simulink model "V2x_TC_CarBreakdownWarning_cs"  (Simulink 7.6)
settings: Solver=ode5  SolverMode=SingleTasking  StartTime=0.0  StopTime=18  FixedStep=1/100  RelTol=1e-3
PreLoadFcn:
  | check_NUTS_defined;
  | 
  | assignin('base',['model_closed_' bdroot],false);addpath('../includes_V2x');
InitFcn:
  | PreScanExperimentInitFcn(bdroot)
StopFcn:
  | PreScanExperimentStopFcn(bdroot)
undefined symbols (not defined in the file or in its folder): acceleration, actorID, actorType, DiscIntNeverNeededParam, GPS_alt, GPS_lat, GPS_long, intmax, lightBarInUse, messageID, Newton, publicActorType, Raphson, rotZ, sigbuilder_block, sireneInUse, trafficLightPriority, turnAdvice, velocity, x_ini_VRML, y_ini_VRML, yawRate, z_ini_VRML
libraries: simulink x61, PreScanSimulinkLibrary x19, PreScanUsefulBlocks x7, simulink_extras x1
(part 10 of 10)

== system V2x_TC_CarBreakdownWarning_cs/Audi_A8_1/vehicle CAM generator/CAM generation/maybe/If Action Subsystem ==
  x [m] : Inport
  y [m] : Inport  Port=2
  z [m] : Inport  Port=3
  rotZ [deg] : Inport  Port=4
  velocity [m/s] : Inport  Port=5
  Action Port : ActionPort  PropagateVarSize=During execution  ActionType=then
  Constant : Constant
  Data Store Write : DataStoreWrite  DataStoreName=CAM_velocity
  Data Store Write1 : DataStoreWrite  DataStoreName=CAM_heading
  Data Store Write2 : DataStoreWrite  DataStoreName=CAM_x
  Data Store Write3 : DataStoreWrite  DataStoreName=CAM_y
  Data Store Write4 : DataStoreWrite  DataStoreName=CAM_z
  Data Store Write5 : DataStoreWrite  DataStoreName=CAM_time
  Digital Clock1 : DigitalClock  SampleTime=0.01
  Out1 : Outport  InitialOutput=0
  wires:
  Constant/1 -> Out1/1
  velocity [m/s]/1 -> Data Store Write/1
  rotZ [deg]/1 -> Data Store Write1/1
  x [m]/1 -> Data Store Write2/1
  y [m]/1 -> Data Store Write3/1
  z [m]/1 -> Data Store Write4/1
  Digital Clock1/1 -> Data Store Write5/1

== system V2x_TC_CarBreakdownWarning_cs/Audi_A8_1/vehicle CAM generator/CAM generation/maybe/If Action Subsystem1 ==
  Action Port : ActionPort  PropagateVarSize=During execution  ActionType=else
  Constant : Constant  Value=0
  Out1 : Outport  InitialOutput=0
  wires:
  Constant/1 -> Out1/1

== system V2x_TC_CarBreakdownWarning_cs/BMW_X5_1/Trajectories/Traj2State1/Traj2State2/MuxState ==
  x [m] : Inport
  y [m] : Inport  Port=2
  z [m] : Inport  Port=3
  dx [m/s] : Inport  Port=4
  dy [m/s] : Inport  Port=5
  dz [m/s] : Inport  Port=6
  R [rad] : Inport  Port=7
  P [rad] : Inport  Port=8
  Y [rad] : Inport  Port=9
  Mux : Mux  Inputs=9
  state : Outport
  wires:
  z [m]/1 -> Mux/3
  y [m]/1 -> Mux/2
  x [m]/1 -> Mux/1
  Y [rad]/1 -> Mux/9
  P [rad]/1 -> Mux/8
  R [rad]/1 -> Mux/7
  dz [m/s]/1 -> Mux/6
  dy [m/s]/1 -> Mux/5
  dx [m/s]/1 -> Mux/4
  Mux/1 -> state/1

== system V2x_TC_CarBreakdownWarning_cs/BMW_X5_1/Trajectories/Traj2State1/Traj2State2/Traj2MuxState_Ext ==
  Traj : Inport
  Terminator{1..9} (9 alike) : Terminator
  demux : Subsystem
  x [m] : Outport
  y [m] : Outport  Port=2
  z [m] : Outport  Port=3
  dx [m/s] : Outport  Port=4
  dy [m/s] : Outport  Port=5
  dz [m/s] : Outport  Port=6
  R [rad] : Outport  Port=7
  P [rad] : Outport  Port=8
  Y [rad] : Outport  Port=9
  wires:
  demux/9(Y) -> Y [rad]/1
  demux/7(R) -> R [rad]/1
  demux/5(vely) -> dy [m/s]/1
  demux/4(velx) -> dx [m/s]/1
  demux/10(velR) -> Terminator4/1
  demux/11(velP) -> Terminator5/1
  demux/12(velY) -> Terminator1/1
  demux/13(accx) -> Terminator8/1
  demux/14(accy) -> Terminator9/1
  demux/15(accz) -> Terminator7/1
  demux/18(accY) -> Terminator2/1
  demux/16(accR) -> Terminator3/1
  demux/17(accP) -> Terminator6/1
  demux/3(z) -> z [m]/1
  Traj/1 -> demux/1(traj)
  demux/6(velz) -> dz [m/s]/1
  demux/1(x) -> x [m]/1
  demux/2(y) -> y [m]/1
  demux/8(P) -> P [rad]/1

== system V2x_TC_CarBreakdownWarning_cs/BMW_X5_1/vehicle CAM generator/CAM generation/maybe/If Action Subsystem ==
  x [m] : Inport
  y [m] : Inport  Port=2
  z [m] : Inport  Port=3
  rotZ [deg] : Inport  Port=4
  velocity [m/s] : Inport  Port=5
  Action Port : ActionPort  PropagateVarSize=During execution  ActionType=then
  Constant : Constant
  Data Store Write : DataStoreWrite  DataStoreName=CAM_velocity
  Data Store Write1 : DataStoreWrite  DataStoreName=CAM_heading
  Data Store Write2 : DataStoreWrite  DataStoreName=CAM_x
  Data Store Write3 : DataStoreWrite  DataStoreName=CAM_y
  Data Store Write4 : DataStoreWrite  DataStoreName=CAM_z
  Data Store Write5 : DataStoreWrite  DataStoreName=CAM_time
  Digital Clock1 : DigitalClock  SampleTime=0.01
  Out1 : Outport  InitialOutput=0
  wires:
  Constant/1 -> Out1/1
  velocity [m/s]/1 -> Data Store Write/1
  rotZ [deg]/1 -> Data Store Write1/1
  x [m]/1 -> Data Store Write2/1
  y [m]/1 -> Data Store Write3/1
  z [m]/1 -> Data Store Write4/1
  Digital Clock1/1 -> Data Store Write5/1

== system V2x_TC_CarBreakdownWarning_cs/BMW_X5_1/vehicle CAM generator/CAM generation/maybe/If Action Subsystem1 ==
  Action Port : ActionPort  PropagateVarSize=During execution  ActionType=else
  Constant : Constant  Value=0
  Out1 : Outport  InitialOutput=0
  wires:
  Constant/1 -> Out1/1

== system V2x_TC_CarBreakdownWarning_cs/Fiat_Bravo_1/Trajectories/Traj2State1/Traj2State2/MuxState ==
  x [m] : Inport
  y [m] : Inport  Port=2
  z [m] : Inport  Port=3
  dx [m/s] : Inport  Port=4
  dy [m/s] : Inport  Port=5
  dz [m/s] : Inport  Port=6
  R [rad] : Inport  Port=7
  P [rad] : Inport  Port=8
  Y [rad] : Inport  Port=9
  Mux : Mux  Inputs=9
  state : Outport
  wires:
  z [m]/1 -> Mux/3
  y [m]/1 -> Mux/2
  x [m]/1 -> Mux/1
  Y [rad]/1 -> Mux/9
  P [rad]/1 -> Mux/8
  R [rad]/1 -> Mux/7
  dz [m/s]/1 -> Mux/6
  dy [m/s]/1 -> Mux/5
  dx [m/s]/1 -> Mux/4
  Mux/1 -> state/1

== system V2x_TC_CarBreakdownWarning_cs/Fiat_Bravo_1/Trajectories/Traj2State1/Traj2State2/Traj2MuxState_Ext ==
  Traj : Inport
  Terminator{1..9} (9 alike) : Terminator
  demux : Subsystem
  x [m] : Outport
  y [m] : Outport  Port=2
  z [m] : Outport  Port=3
  dx [m/s] : Outport  Port=4
  dy [m/s] : Outport  Port=5
  dz [m/s] : Outport  Port=6
  R [rad] : Outport  Port=7
  P [rad] : Outport  Port=8
  Y [rad] : Outport  Port=9
  wires:
  demux/9(Y) -> Y [rad]/1
  demux/7(R) -> R [rad]/1
  demux/5(vely) -> dy [m/s]/1
  demux/4(velx) -> dx [m/s]/1
  demux/10(velR) -> Terminator4/1
  demux/11(velP) -> Terminator5/1
  demux/12(velY) -> Terminator1/1
  demux/13(accx) -> Terminator8/1
  demux/14(accy) -> Terminator9/1
  demux/15(accz) -> Terminator7/1
  demux/18(accY) -> Terminator2/1
  demux/16(accR) -> Terminator3/1
  demux/17(accP) -> Terminator6/1
  demux/3(z) -> z [m]/1
  Traj/1 -> demux/1(traj)
  demux/6(velz) -> dz [m/s]/1
  demux/1(x) -> x [m]/1
  demux/2(y) -> y [m]/1
  demux/8(P) -> P [rad]/1

== system V2x_TC_CarBreakdownWarning_cs/Fiat_Bravo_1/vehicle CAM generator/CAM generation/maybe/If Action Subsystem ==
  x [m] : Inport
  y [m] : Inport  Port=2
  z [m] : Inport  Port=3
  rotZ [deg] : Inport  Port=4
  velocity [m/s] : Inport  Port=5
  Action Port : ActionPort  PropagateVarSize=During execution  ActionType=then
  Constant : Constant
  Data Store Write : DataStoreWrite  DataStoreName=CAM_velocity
  Data Store Write1 : DataStoreWrite  DataStoreName=CAM_heading
  Data Store Write2 : DataStoreWrite  DataStoreName=CAM_x
  Data Store Write3 : DataStoreWrite  DataStoreName=CAM_y
  Data Store Write4 : DataStoreWrite  DataStoreName=CAM_z
  Data Store Write5 : DataStoreWrite  DataStoreName=CAM_time
  Digital Clock1 : DigitalClock  SampleTime=0.01
  Out1 : Outport  InitialOutput=0
  wires:
  Constant/1 -> Out1/1
  velocity [m/s]/1 -> Data Store Write/1
  rotZ [deg]/1 -> Data Store Write1/1
  x [m]/1 -> Data Store Write2/1
  y [m]/1 -> Data Store Write3/1
  z [m]/1 -> Data Store Write4/1
  Digital Clock1/1 -> Data Store Write5/1

== system V2x_TC_CarBreakdownWarning_cs/Fiat_Bravo_1/vehicle CAM generator/CAM generation/maybe/If Action Subsystem1 ==
  Action Port : ActionPort  PropagateVarSize=During execution  ActionType=else
  Constant : Constant  Value=0
  Out1 : Outport  InitialOutput=0
  wires:
  Constant/1 -> Out1/1

== system V2x_TC_CarBreakdownWarning_cs/Toyota_Previa_1/vehicle CAM generator/CAM generation/maybe/If Action Subsystem ==
  x [m] : Inport
  y [m] : Inport  Port=2
  z [m] : Inport  Port=3
  rotZ [deg] : Inport  Port=4
  velocity [m/s] : Inport  Port=5
  Action Port : ActionPort  PropagateVarSize=During execution  ActionType=then
  Constant : Constant
  Data Store Write : DataStoreWrite  DataStoreName=CAM_velocity
  Data Store Write1 : DataStoreWrite  DataStoreName=CAM_heading
  Data Store Write2 : DataStoreWrite  DataStoreName=CAM_x
  Data Store Write3 : DataStoreWrite  DataStoreName=CAM_y
  Data Store Write4 : DataStoreWrite  DataStoreName=CAM_z
  Data Store Write5 : DataStoreWrite  DataStoreName=CAM_time
  Digital Clock1 : DigitalClock  SampleTime=0.01
  Out1 : Outport  InitialOutput=0
  wires:
  Constant/1 -> Out1/1
  velocity [m/s]/1 -> Data Store Write/1
  rotZ [deg]/1 -> Data Store Write1/1
  x [m]/1 -> Data Store Write2/1
  y [m]/1 -> Data Store Write3/1
  z [m]/1 -> Data Store Write4/1
  Digital Clock1/1 -> Data Store Write5/1

== system V2x_TC_CarBreakdownWarning_cs/Toyota_Previa_1/vehicle CAM generator/CAM generation/maybe/If Action Subsystem1 ==
  Action Port : ActionPort  PropagateVarSize=During execution  ActionType=else
  Constant : Constant  Value=0
  Out1 : Outport  InitialOutput=0
  wires:
  Constant/1 -> Out1/1

== system V2x_TC_CarBreakdownWarning_cs/Audi_A8_1/Traffic Controller/Intersection warning controller/Enabled Subsystem/Intersection/Closest crossing selection ==
  crossingType : Inport
  host GPS lat : Inport  Port=2
  host GPS long : Inport  Port=3
  host GPS alt : Inport  Port=4
  GPS lat : Inport  Port=5
  GPS long : Inport  Port=6
  GPS alt : Inport  Port=7
  crossing detection range : Inport  Port=8
  GPS alt1 : InportShadow  Port=7
  GPS lat1 : InportShadow  Port=5
  GPS long1 : InportShadow  Port=6
  GPS to XYZ difference (vectorized) : Subsystem
  If : If  NumInputs=2  IfExpression=u1 ~= u2
  If Action Subsystem : Subsystem  TreatAsAtomicUnit=on
  If Action Subsystem1 : Subsystem  TreatAsAtomicUnit=on
  Logical Operator : Logic  AllPortsSameDT=off  OutDataTypeStr=boolean
  Merge : Merge
  Merge1 : Merge
  Merge2 : Merge
  MinMax : MinMax
  Product : Product  RndMeth=Zero
  Relational Operator : RelationalOperator  Operator=<  OutDataTypeStr=boolean
  Switch : Switch  Criteria=u2 > Threshold
  crossing GPS lat : Outport
  crossing GPS long : Outport  Port=2
  crossing GPS alt : Outport  Port=3
  wires:
  GPS to XYZ difference (vectorized)/1(dist_sq) -> Relational Operator/1, Switch/1, If Action Subsystem/2(dist_sq)
  crossing detection range/1 -> Product/2, Product/1
  Product/1 -> Relational Operator/2, Switch/3, If/2
  Relational Operator/1 -> Logical Operator/1
  crossingType/1 -> Logical Operator/2
  Logical Operator/1 -> Switch/2
  Switch/1 -> MinMax/1
  MinMax/1 -> If Action Subsystem/1(min), If/1
  host GPS lat/1 -> GPS to XYZ difference (vectorized)/1(hostLat)
  host GPS long/1 -> GPS to XYZ difference (vectorized)/2(hostLong)
  host GPS alt/1 -> GPS to XYZ difference (vectorized)/3(hostAlt)
  GPS lat/1 -> GPS to XYZ difference (vectorized)/4(lat)
  GPS long/1 -> GPS to XYZ difference (vectorized)/5(long)
  GPS alt/1 -> GPS to XYZ difference (vectorized)/6(alt)
  If/1 -> If Action Subsystem/Action
  If/2 -> If Action Subsystem1/Action
  GPS lat1/1 -> If Action Subsystem/3(GPS lat1)
  GPS long1/1 -> If Action Subsystem/4(GPS long1)
  GPS alt1/1 -> If Action Subsystem/5(GPS alt1)
  If Action Subsystem/1(GPS lat) -> Merge/1
  If Action Subsystem/2(GPS long) -> Merge2/1
  If Action Subsystem/3(GPS alt) -> Merge1/1
  If Action Subsystem1/1(GPS lat) -> Merge/2
  If Action Subsystem1/2(GPS long) -> Merge2/2
  If Action Subsystem1/3(GPS alt) -> Merge1/2
  Merge2/1 -> crossing GPS long/1
  Merge/1 -> crossing GPS lat/1
  Merge1/1 -> crossing GPS alt/1

== system V2x_TC_CarBreakdownWarning_cs/Audi_A8_1/Traffic Controller/Intersection warning controller/Enabled Subsystem/Intersection/GPS to XYZ difference (vectorized) ==
  hostLat : Inport
  hostLong : Inport  Port=2
  hostAlt : Inport  Port=3
  lat : Inport  Port=4
  long : Inport  Port=5
  alt : Inport  Port=6
  Add : Sum  Inputs=+-
  Add1 : Sum  Inputs=+-
  Add2 : Sum  Inputs=+-
  Product1 : Product  RndMeth=Zero
  Product2 : Product  RndMeth=Zero
  d2r : Gain  Gain=pi/180
  d2r1 : Gain  Gain=pi/180
  mean Earth radius (latitudal) : Constant  Value=6335439.8775
  mean Earth radius (longitudal) : Constant  Value=6378137.55
  dX : Outport
  dY : Outport  Port=2
  dZ : Outport  Port=3
  wires:
  lat/1 -> Add/1
  hostLat/1 -> Add/2
  long/1 -> Add1/1
  hostLong/1 -> Add1/2
  alt/1 -> Add2/1
  hostAlt/1 -> Add2/2
  Add/1 -> d2r/1
  Add1/1 -> d2r1/1
  d2r/1 -> Product2/1
  d2r1/1 -> Product1/1
  mean Earth radius (longitudal)/1 -> Product1/2
  mean Earth radius (latitudal)/1 -> Product2/2
  Product2/1 -> dY/1
  Product1/1 -> dX/1
  Add2/1 -> dZ/1

== system V2x_TC_CarBreakdownWarning_cs/Audi_A8_1/Traffic Controller/Intersection warning controller/Enabled Subsystem/Intersection/Intersection collision warning controller ==
  actorType : Inport
  hostTurnAdvice : Inport  Port=2
  crossing detection range : Inport  Port=3
  target intention : Inport  Port=4
  target velocity : Inport  Port=5
  target range : Inport  Port=6
  target angle : Inport  Port=7
  target heading : Inport  Port=8
  For Each Subsystem : Subsystem  TreatAsAtomicUnit=on
  Logical Operator : Logic  Operator=OR  Inputs=1  AllPortsSameDT=off  OutDataTypeStr=boolean
  Logical Operator1 : Logic  Operator=OR  Inputs=1  AllPortsSameDT=off  OutDataTypeStr=boolean
  Logical Operator2 : Logic  Operator=OR  Inputs=1  AllPortsSameDT=off  OutDataTypeStr=boolean
  host intention translation : Subsystem
  warning left lane : Outport
  warning straight lane : Outport  Port=2
  warning right lane : Outport  Port=3
  wires:
  hostTurnAdvice/1 -> host intention translation/1(host intention)
  For Each Subsystem/1(warning left lane) -> Logical Operator/1
  For Each Subsystem/2(warning straight lane) -> Logical Operator1/1
  For Each Subsystem/3(warning right lane) -> Logical Operator2/1
  actorType/1 -> For Each Subsystem/1(actorType)
  host intention translation/1(WM) -> For Each Subsystem/2(WM)
  crossing detection range/1 -> For Each Subsystem/3(Rcross)
  target range/1 -> For Each Subsystem/4(target range)
  target angle/1 -> For Each Subsystem/5(target angle)
  target intention/1 -> For Each Subsystem/6(target intention)
  target heading/1 -> For Each Subsystem/7(target heading)
  Logical Operator/1 -> warning left lane/1
  Logical Operator1/1 -> warning straight lane/1
  Logical Operator2/1 -> warning right lane/1
  target velocity/1 -> For Each Subsystem/8(targetVelocity)

== system V2x_TC_CarBreakdownWarning_cs/Audi_A8_1/Traffic Controller/Intersection warning controller/Enabled Subsystem/Intersection/cartesian 2 cylindrical ==
  dX : Inport
  dY : Inport  Port=2
  hostRotZ : Inport  Port=3
  Add : Sum  Inputs=+-
  Complex to Magnitude-Angle1 : ComplexToMagnitudeAngle
  Real-Imag to Complex1 : RealImagToComplex
  r2d : Gain  Gain=180/pi
  range : Outport
  angle : Outport  Port=2
  wires:
  Real-Imag to Complex1/1 -> Complex to Magnitude-Angle1/1
  dX/1 -> Real-Imag to Complex1/1
  Complex to Magnitude-Angle1/1 -> range/1  "range"
  dY/1 -> Real-Imag to Complex1/2
  Complex to Magnitude-Angle1/2 -> r2d/1  "angle"
  r2d/1 -> Add/1
  hostRotZ/1 -> Add/2
  Add/1 -> angle/1

== system V2x_TC_CarBreakdownWarning_cs/Audi_A8_1/Traffic Controller/Intersection warning controller/Enabled Subsystem/Intersection/relative heading ==
  rotZ : Inport
  hostRotZ : Inport  Port=2
  Add : Sum  Inputs=+-
  Constant : Constant  Value=360
  Math Function : Math  Operator=mod  SaturateOnIntegerOverflow=on
  dRotZ : Outport
  wires:
  Constant/1 -> Math Function/2
  rotZ/1 -> Add/1
  hostRotZ/1 -> Add/2
  Add/1 -> Math Function/1
  Math Function/1 -> dRotZ/1

== system V2x_TC_CarBreakdownWarning_cs/Audi_A8_1/Traffic Controller/Road accident detection controller/Compute distance to road accident/If Action Subsystem/GPS to distance ==
  hostLat : Inport
  hostLong : Inport  Port=2
  hostAlt : Inport  Port=3
  lat : Inport  Port=4
  long : Inport  Port=5
  alt : Inport  Port=6
  Add : Sum  Inputs=+-
  Add1 : Sum  Inputs=+-
  Add2 : Sum  Inputs=+-
  Add3 : Sum  Inputs=+++
  Product{,1..4} (5 alike) : Product  RndMeth=Zero
  Sqrt : Sqrt  AlgorithmType=Newton-Raphson  SaturateOnIntegerOverflow=on
  d2r : Gain  Gain=pi/180
  d2r1 : Gain  Gain=pi/180
  mean Earth radius (latitudal) : Constant  Value=6335439.8775
  mean Earth radius (longitudal) : Constant  Value=6378137.55
  dist : Outport
  wires:
  lat/1 -> Add/1
  hostLat/1 -> Add/2
  long/1 -> Add1/1
  hostLong/1 -> Add1/2
  alt/1 -> Add2/1
  hostAlt/1 -> Add2/2
  Add/1 -> d2r/1
  Add1/1 -> d2r1/1
  d2r/1 -> Product2/1
  d2r1/1 -> Product1/1
  mean Earth radius (longitudal)/1 -> Product1/2
  mean Earth radius (latitudal)/1 -> Product2/2
  Product2/1 -> Product/1, Product/2
  Product1/1 -> Product3/1, Product3/2
  Add2/1 -> Product4/2, Product4/1
  Product/1 -> Add3/1
  Product3/1 -> Add3/2
  Product4/1 -> Add3/3
  Add3/1 -> Sqrt/1
  Sqrt/1 -> dist/1

== system V2x_TC_CarBreakdownWarning_cs/Audi_A8_1/Traffic Controller/Traffic signs and  traffic lights controller/Enabled Subsystem/distance condition/If Action Subsystem ==
  d2 : Inport
  v2 : Inport  Port=2
  Action Port : ActionPort  PropagateVarSize=During execution  ActionType=then
  Divide : Product  Inputs=*/
  t2 : Outport
  wires:
  Divide/1 -> t2/1
  v2/1 -> Divide/2
  d2/1 -> Divide/1

== system V2x_TC_CarBreakdownWarning_cs/Audi_A8_1/Traffic Controller/Traffic signs and  traffic lights controller/Enabled Subsystem/distance condition/If Action Subsystem1 ==
  headway time : Inport
  d2 : Inport  Port=2
  Action Port : ActionPort  PropagateVarSize=During execution  ActionType=else
  Add : Sum
  Gain : Gain  Gain=0
  t2 : Outport
  wires:
  Add/1 -> t2/1
  headway time/1 -> Add/2
  Gain/1 -> Add/1
  d2/1 -> Gain/1

== system V2x_TC_CarBreakdownWarning_cs/Audi_A8_1/Traffic Controller/Traffic signs and  traffic lights controller/Enabled Subsystem/major object selection lights/If Action Subsystem ==
  cond : Inport
  messagesID : Inport  Port=2
  traffic lights priorities : Inport  Port=3
  Action Port : ActionPort  PropagateVarSize=During execution  ActionType=then
  Reshape1 : Reshape  OutputDimensionality=Column vector (2-D)
  Reshape2 : Reshape  OutputDimensionality=Column vector (2-D)
  Reshape3 : Reshape  OutputDimensionality=Column vector (2-D)
  Selector : Selector  NumberOfDimensions=2  InputPortWidth=3  IndexOptions=Index vector (port),Index vector (dialog)  Indices=[1 3],1  OutputSizes=1,1
  Selector1 : Selector  NumberOfDimensions=2  InputPortWidth=3  IndexOptions=Index vector (port),Index vector (dialog)  Indices=[1 3],1  OutputSizes=1,1
  While Iterator Subsystem : Subsystem  TreatAsAtomicUnit=on
  Message : Outport  InitialOutput=0
  Priority : Outport  Port=2  InitialOutput=0
  wires:
  Selector1/1 -> Priority/1
  Reshape3/1 -> Selector1/1
  traffic lights priorities/1 -> Reshape3/1
  messagesID/1 -> Reshape2/1
  While Iterator Subsystem/1(idx) -> Selector1/2, Selector/2
  Reshape2/1 -> Selector/1
  Reshape1/1 -> While Iterator Subsystem/1(cond)
  Selector/1 -> Message/1
  cond/1 -> Reshape1/1

== system V2x_TC_CarBreakdownWarning_cs/Audi_A8_1/Traffic Controller/Traffic signs and  traffic lights controller/Enabled Subsystem/major object selection lights/If Action Subsystem1 ==
  Action Port : ActionPort  PropagateVarSize=During execution  ActionType=else
  Constant1 : Constant  Value=0
  Constant2 : Constant  Value=0
  Message : Outport  InitialOutput=0
  Priority : Outport  Port=2  InitialOutput=0
  wires:
  Constant2/1 -> Priority/1
  Constant1/1 -> Message/1

== system V2x_TC_CarBreakdownWarning_cs/Audi_A8_1/Traffic Controller/Traffic signs and  traffic lights controller/Enabled Subsystem/major object selection lights/Traffic Lights Warning ==
  trafficLightPriority : Inport
  Data Type Conversion : DataTypeConversion
  Logical Operator : Logic  Operator=OR  AllPortsSameDT=off  OutDataTypeStr=boolean
  if Orange light : simulink/Logic and Bit Operations/Compare To Constant  SystemSampleTime=-1  relop===  const=2  LogicOutDataTypeMode=uint8  ZeroCross=off
  if Red light : simulink/Logic and Bit Operations/Compare To Constant  SystemSampleTime=-1  relop===  const=1  LogicOutDataTypeMode=uint8  ZeroCross=off
  Warning : Outport
  wires:
  trafficLightPriority/1 -> if Orange light/1, if Red light/1
  Data Type Conversion/1 -> Warning/1
  Logical Operator/1 -> Data Type Conversion/1
  if Red light/1 -> Logical Operator/2
  if Orange light/1 -> Logical Operator/1

== system V2x_TC_CarBreakdownWarning_cs/Audi_A8_1/Traffic Controller/Traffic signs and  traffic lights controller/Enabled Subsystem/major object selection signs/If Action Subsystem ==
  cond : Inport
  messagesID : Inport  Port=2
  hostVelocity : Inport  Port=3
  Action Port : ActionPort  PropagateVarSize=During execution  ActionType=then
  Reshape1 : Reshape  OutputDimensionality=Column vector (2-D)
  Reshape2 : Reshape  OutputDimensionality=Column vector (2-D)
  Selector : Selector  NumberOfDimensions=2  InputPortWidth=3  IndexOptions=Index vector (port),Index vector (dialog)  Indices=[1 3],1  OutputSizes=1,1
  Selector1 : Selector  NumberOfDimensions=2  InputPortWidth=3  IndexOptions=Index vector (port),Index vector (dialog)  Indices=[1 3],1  OutputSizes=1,1
  Traffic signs warning : Subsystem
  While Iterator Subsystem : Subsystem  TreatAsAtomicUnit=on
  Warning : Outport
  Message : Outport  Port=2  InitialOutput=0
  wires:
  Selector1/1 -> Traffic signs warning/1(MessageID)
  Traffic signs warning/1(Warning) -> Warning/1
  hostVelocity/1 -> Traffic signs warning/2(hostVelocity)
  messagesID/1 -> Reshape2/1
  While Iterator Subsystem/1(idx) -> Selector1/2, Selector/2
  Reshape2/1 -> Selector1/1, Selector/1
  Reshape1/1 -> While Iterator Subsystem/1(cond)
  Selector/1 -> Message/1
  cond/1 -> Reshape1/1

== system V2x_TC_CarBreakdownWarning_cs/Audi_A8_1/Traffic Controller/Traffic signs and  traffic lights controller/Enabled Subsystem/major object selection signs/If Action Subsystem1 ==
  Action Port : ActionPort  PropagateVarSize=During execution  ActionType=else
  Constant1 : Constant  Value=0
  Constant2 : Constant  Value=0
  Warning : Outport  InitialOutput=0
  Message : Outport  Port=2  InitialOutput=0
  wires:
  Constant2/1 -> Warning/1
  Constant1/1 -> Message/1

== system V2x_TC_CarBreakdownWarning_cs/Audi_A8_1/Traffic Controller/Traffic signs and  traffic lights controller/Enabled Subsystem/orientation condition/to local reference system ==
  rotZ : Inport
  dX : Inport  Port=2
  dY : Inport  Port=3
  Add : Sum
  Add1 : Sum  Inputs=+-
  Product{,1..3} (4 alike) : Product  RndMeth=Zero
  Trigonometric Function : Trigonometry
  Trigonometric Function1 : Trigonometry  Operator=cos
  dy : Outport
  dx : Outport  Port=2
  wires:
  Add1/1 -> dy/1
  Add/1 -> dx/1
  Product3/1 -> Add1/2
  Product2/1 -> Add1/1
  Product/1 -> Add/2
  Product1/1 -> Add/1
  dY/1 -> Product2/2, Product1/2
  Trigonometric Function/1 -> Product3/1, Product1/1
  dX/1 -> Product3/2, Product/2
  Trigonometric Function1/1 -> Product2/1, Product/1
  rotZ/1 -> Trigonometric Function1/1, Trigonometric Function/1

== system V2x_TC_CarBreakdownWarning_cs/Audi_A8_1/Traffic Controller/Traffic signs and  traffic lights controller/Enabled Subsystem/right road side condition/to local reference system ==
  rotZ : Inport
  dX : Inport  Port=2
  dY : Inport  Port=3
  Add1 : Sum  Inputs=+-
  Product2 : Product  RndMeth=Zero
  Product3 : Product  RndMeth=Zero
  Trigonometric Function : Trigonometry
  Trigonometric Function1 : Trigonometry  Operator=cos
  dy : Outport
  wires:
  rotZ/1 -> Trigonometric Function/1, Trigonometric Function1/1
  Trigonometric Function1/1 -> Product2/1
  dX/1 -> Product3/2
  Trigonometric Function/1 -> Product3/1
  dY/1 -> Product2/2
  Product2/1 -> Add1/1
  Product3/1 -> Add1/2
  Add1/1 -> dy/1

== system V2x_TC_CarBreakdownWarning_cs/Audi_A8_1/Trajectories/Traj2State1/Traj2State2/Traj2MuxState_Ext/demux ==
  traj : Inport
  Demux : Demux  Outputs=18
  x : Outport
  y : Outport  Port=2
  z : Outport  Port=3
  velx : Outport  Port=4
  vely : Outport  Port=5
  velz : Outport  Port=6
  R : Outport  Port=7
  P : Outport  Port=8
  Y : Outport  Port=9
  velR : Outport  Port=10
  velP : Outport  Port=11
  velY : Outport  Port=12
  accx : Outport  Port=13
  accy : Outport  Port=14
  accz : Outport  Port=15
  accR : Outport  Port=16
  accP : Outport  Port=17
  accY : Outport  Port=18
  wires:
  Demux/18 -> accY/1
  Demux/17 -> accP/1
  Demux/16 -> accR/1
  Demux/15 -> accz/1
  Demux/14 -> accy/1
  Demux/13 -> accx/1
  Demux/12 -> velY/1
  Demux/11 -> velP/1
  Demux/10 -> velR/1
  Demux/9 -> velz/1
  Demux/8 -> vely/1
  Demux/7 -> velx/1
  Demux/6 -> Y/1
  Demux/5 -> P/1
  traj/1 -> Demux/1
  Demux/4 -> R/1
  Demux/3 -> z/1
  Demux/2 -> y/1
  Demux/1 -> x/1

== system V2x_TC_CarBreakdownWarning_cs/Audi_A8_1/Trajectories/Traj2State2/Traj2State2/Traj2MuxState_Ext/demux ==
  traj : Inport
  Demux : Demux  Outputs=18
  x : Outport
  y : Outport  Port=2
  z : Outport  Port=3
  velx : Outport  Port=4
  vely : Outport  Port=5
  velz : Outport  Port=6
  R : Outport  Port=7
  P : Outport  Port=8
  Y : Outport  Port=9
  velR : Outport  Port=10
  velP : Outport  Port=11
  velY : Outport  Port=12
  accx : Outport  Port=13
  accy : Outport  Port=14
  accz : Outport  Port=15
  accR : Outport  Port=16
  accP : Outport  Port=17
  accY : Outport  Port=18
  wires:
  Demux/18 -> accY/1
  Demux/17 -> accP/1
  Demux/16 -> accR/1
  Demux/15 -> accz/1
  Demux/14 -> accy/1
  Demux/13 -> accx/1
  Demux/12 -> velY/1
  Demux/11 -> velP/1
  Demux/10 -> velR/1
  Demux/9 -> velz/1
  Demux/8 -> vely/1
  Demux/7 -> velx/1
  Demux/6 -> Y/1
  Demux/5 -> P/1
  traj/1 -> Demux/1
  Demux/4 -> R/1
  Demux/3 -> z/1
  Demux/2 -> y/1
  Demux/1 -> x/1

== system V2x_TC_CarBreakdownWarning_cs/BMW_X5_1/Trajectories/Traj2State1/Traj2State2/Traj2MuxState_Ext/demux ==
  traj : Inport
  Demux : Demux  Outputs=18
  x : Outport
  y : Outport  Port=2
  z : Outport  Port=3
  velx : Outport  Port=4
  vely : Outport  Port=5
  velz : Outport  Port=6
  R : Outport  Port=7
  P : Outport  Port=8
  Y : Outport  Port=9
  velR : Outport  Port=10
  velP : Outport  Port=11
  velY : Outport  Port=12
  accx : Outport  Port=13
  accy : Outport  Port=14
  accz : Outport  Port=15
  accR : Outport  Port=16
  accP : Outport  Port=17
  accY : Outport  Port=18
  wires:
  Demux/18 -> accY/1
  Demux/17 -> accP/1
  Demux/16 -> accR/1
  Demux/15 -> accz/1
  Demux/14 -> accy/1
  Demux/13 -> accx/1
  Demux/12 -> velY/1
  Demux/11 -> velP/1
  Demux/10 -> velR/1
  Demux/9 -> velz/1
  Demux/8 -> vely/1
  Demux/7 -> velx/1
  Demux/6 -> Y/1
  Demux/5 -> P/1
  traj/1 -> Demux/1
  Demux/4 -> R/1
  Demux/3 -> z/1
  Demux/2 -> y/1
  Demux/1 -> x/1

== system V2x_TC_CarBreakdownWarning_cs/Fiat_Bravo_1/Trajectories/Traj2State1/Traj2State2/Traj2MuxState_Ext/demux ==
  traj : Inport
  Demux : Demux  Outputs=18
  x : Outport
  y : Outport  Port=2
  z : Outport  Port=3
  velx : Outport  Port=4
  vely : Outport  Port=5
  velz : Outport  Port=6
  R : Outport  Port=7
  P : Outport  Port=8
  Y : Outport  Port=9
  velR : Outport  Port=10
  velP : Outport  Port=11
  velY : Outport  Port=12
  accx : Outport  Port=13
  accy : Outport  Port=14
  accz : Outport  Port=15
  accR : Outport  Port=16
  accP : Outport  Port=17
  accY : Outport  Port=18
  wires:
  Demux/18 -> accY/1
  Demux/17 -> accP/1
  Demux/16 -> accR/1
  Demux/15 -> accz/1
  Demux/14 -> accy/1
  Demux/13 -> accx/1
  Demux/12 -> velY/1
  Demux/11 -> velP/1
  Demux/10 -> velR/1
  Demux/9 -> velz/1
  Demux/8 -> vely/1
  Demux/7 -> velx/1
  Demux/6 -> Y/1
  Demux/5 -> P/1
  traj/1 -> Demux/1
  Demux/4 -> R/1
  Demux/3 -> z/1
  Demux/2 -> y/1
  Demux/1 -> x/1

== system V2x_TC_CarBreakdownWarning_cs/Audi_A8_1/Traffic Controller/Intersection warning controller/Enabled Subsystem/Intersection/Closest crossing selection/GPS to XYZ difference (vectorized) ==
  hostLat : Inport
  hostLong : Inport  Port=2
  hostAlt : Inport  Port=3
  lat : Inport  Port=4
  long : Inport  Port=5
  alt : Inport  Port=6
  Add : Sum  Inputs=+-
  Add1 : Sum  Inputs=+-
  Add2 : Sum  Inputs=+-
  Add3 : Sum  Inputs=+++
  Product{,1..4} (5 alike) : Product  RndMeth=Zero
  d2r : Gain  Gain=pi/180
  d2r1 : Gain  Gain=pi/180
  mean Earth radius (latitudal) : Constant  Value=6335439.8775
  mean Earth radius (longitudal) : Constant  Value=6378137.55
  dist_sq : Outport
  wires:
  lat/1 -> Add/1
  hostLat/1 -> Add/2
  long/1 -> Add1/1
  hostLong/1 -> Add1/2
  alt/1 -> Add2/1
  hostAlt/1 -> Add2/2
  Add/1 -> d2r/1
  Add1/1 -> d2r1/1
  d2r/1 -> Product2/1
  d2r1/1 -> Product1/1
  mean Earth radius (longitudal)/1 -> Product1/2
  mean Earth radius (latitudal)/1 -> Product2/2
  Product2/1 -> Product/1, Product/2
  Product1/1 -> Product3/1, Product3/2
  Add2/1 -> Product4/2, Product4/1
  Product/1 -> Add3/1
  Product3/1 -> Add3/2
  Product4/1 -> Add3/3
  Add3/1 -> dist_sq/1

== system V2x_TC_CarBreakdownWarning_cs/Audi_A8_1/Traffic Controller/Intersection warning controller/Enabled Subsystem/Intersection/Closest crossing selection/If Action Subsystem ==
  min : Inport
  dist_sq : Inport  Port=2
  GPS lat1 : Inport  Port=3
  GPS long1 : Inport  Port=4
  GPS alt1 : Inport  Port=5
  Action Port : ActionPort  PropagateVarSize=During execution  ActionType=then
  Product7 : Product  RndMeth=Zero
  Product8 : Product  RndMeth=Zero
  Product9 : Product  RndMeth=Zero
  Relational Operator3 : RelationalOperator  Operator===  OutDataTypeStr=boolean
  Sum6 : Sum  Inputs=+
  Sum7 : Sum  Inputs=+
  Sum8 : Sum  Inputs=+
  GPS lat : Outport  InitialOutput=0
  GPS long : Outport  Port=2  InitialOutput=0
  GPS alt : Outport  Port=3  InitialOutput=0
  wires:
  min/1 -> Relational Operator3/1
  dist_sq/1 -> Relational Operator3/2
  Relational Operator3/1 -> Product7/1, Product8/1, Product9/1
  GPS lat1/1 -> Product7/2
  GPS long1/1 -> Product8/2
  GPS alt1/1 -> Product9/2
  Product7/1 -> Sum6/1
  Product8/1 -> Sum7/1
  Product9/1 -> Sum8/1
  Sum6/1 -> GPS lat/1
  Sum7/1 -> GPS long/1
  Sum8/1 -> GPS alt/1

== system V2x_TC_CarBreakdownWarning_cs/Audi_A8_1/Traffic Controller/Intersection warning controller/Enabled Subsystem/Intersection/Closest crossing selection/If Action Subsystem1 ==
  Action Port : ActionPort  PropagateVarSize=During execution  ActionType=else
  Constant : Constant  Value=0
  Constant1 : Constant  Value=0
  Constant2 : Constant  Value=0
  GPS lat : Outport  InitialOutput=0
  GPS long : Outport  Port=2  InitialOutput=0
  GPS alt : Outport  Port=3  InitialOutput=0
  wires:
  Constant/1 -> GPS lat/1
  Constant1/1 -> GPS long/1
  Constant2/1 -> GPS alt/1

== system V2x_TC_CarBreakdownWarning_cs/Audi_A8_1/Traffic Controller/Intersection warning controller/Enabled Subsystem/Intersection/Intersection collision warning controller/For Each Subsystem ==
  actorType : Inport  PortDimensions=1  Partition=on  PartitionDimension=1  PartitionWidth=1
  WM : Inport  Port=2  Partition=off
  Rcross : Inport  Port=3  Partition=off
  target range : Inport  Port=4  Partition=on  PartitionDimension=1  PartitionWidth=1
  target angle : Inport  Port=5  Partition=on  PartitionDimension=1  PartitionWidth=1
  target intention : Inport  Port=6  Partition=on  PartitionDimension=1  PartitionWidth=1
  target heading : Inport  Port=7  Partition=on  PartitionDimension=1  PartitionWidth=1
  targetVelocity : Inport  Port=8  PortDimensions=1  Partition=on  PartitionDimension=1  PartitionWidth=1
  For Each : ForEach  DisableCoverage=on  IndexMode=One-based
  If : If  NumInputs=2  IfExpression=(u1==1 | u1==2 | u1 ==3) & (u2~=0)
  If Action Subsystem : Subsystem  TreatAsAtomicUnit=on
  If Action Subsystem1 : Subsystem  TreatAsAtomicUnit=on
  Merge : Merge
  Merge1 : Merge
  Merge2 : Merge
  warning left lane : Outport  ConcatenationDimension=1
  warning straight lane : Outport  Port=2  ConcatenationDimension=1
  warning right lane : Outport  Port=3  ConcatenationDimension=1
  wires:
  actorType/1 -> If/1
  If/1 -> If Action Subsystem/Action
  If/2 -> If Action Subsystem1/Action
  WM/1 -> If Action Subsystem/1(WM)
  Rcross/1 -> If Action Subsystem/2(Rcross)
  target range/1 -> If Action Subsystem/3(target range)
  target angle/1 -> If Action Subsystem/4(target angle)
  target intention/1 -> If Action Subsystem/5(target intention)
  target heading/1 -> If Action Subsystem/6(target heading)
  If Action Subsystem/1(warning left lane) -> Merge/1
  If Action Subsystem/2(warning straight lane) -> Merge1/1
  If Action Subsystem/3(warning right lane) -> Merge2/1
  If Action Subsystem1/1(warning left lane) -> Merge/2
  If Action Subsystem1/2(warning straight lane) -> Merge1/2
  If Action Subsystem1/3(warning right lane) -> Merge2/2
  Merge/1 -> warning left lane/1
  Merge1/1 -> warning straight lane/1
  Merge2/1 -> warning right lane/1
  targetVelocity/1 -> If/2

== system V2x_TC_CarBreakdownWarning_cs/Audi_A8_1/Traffic Controller/Intersection warning controller/Enabled Subsystem/Intersection/Intersection collision warning controller/host intention translation ==
  host intention : Inport
  Bias : Bias  Bias=2
  Multiport Switch : MultiPortSwitch  zeroidx=off
  left_turning : Constant  Value=[0 1 1 1 1 1 0 1 1]
  right_turning : Constant  Value=[0 1 0 0 0 1 0 0 0]
  straight : Constant  Value=[0 1 1 0 0 1 1 1 1]
  WM : Outport
  wires:
  right_turning/1 -> Multiport Switch/4
  straight/1 -> Multiport Switch/3
  left_turning/1 -> Multiport Switch/2
  host intention/1 -> Bias/1
  Bias/1 -> Multiport Switch/1
  Multiport Switch/1 -> WM/1

== system V2x_TC_CarBreakdownWarning_cs/Audi_A8_1/Traffic Controller/Traffic signs and  traffic lights controller/Enabled Subsystem/major object selection lights/If Action Subsystem/While Iterator Subsystem ==
  cond : Inport
  Compare To Zero : simulink/Logic and Bit Operations/Compare To Zero  SystemSampleTime=-1  relop===  LogicOutDataTypeMode=uint8  ZeroCross=off
  Selector : Selector  NumberOfDimensions=2  InputPortWidth=3  IndexOptions=Index vector (port),Index vector (dialog)  Indices=[1 3],1  OutputSizes=1,1
  While Iterator : WhileIterator  MaxIters=-1  WhileBlockType=do-while  ShowIterationPort=on  OutputDataType=double
  idx : Outport
  wires:
  Selector/1 -> Compare To Zero/1
  cond/1 -> Selector/1
  While Iterator/1 -> idx/1, Selector/2
  Compare To Zero/1 -> While Iterator/1

== system V2x_TC_CarBreakdownWarning_cs/Audi_A8_1/Traffic Controller/Traffic signs and  traffic lights controller/Enabled Subsystem/major object selection signs/If Action Subsystem/Traffic signs warning ==
  MessageID : Inport
  hostVelocity : Inport  Port=2
  Compare To Zero : simulink/Logic and Bit Operations/Compare To Zero  SystemSampleTime=-1  relop=>  LogicOutDataTypeMode=uint8  ZeroCross=off
  Data Type Conversion : DataTypeConversion
  Gain : Gain  Gain=3.6
  Logical Operator : Logic  AllPortsSameDT=off  OutDataTypeStr=boolean
  Relational Operator : RelationalOperator  Operator=<  OutDataTypeStr=boolean
  message to speed limit conversion : Bias  Bias=-1000
  Warning : Outport
  wires:
  Logical Operator/1 -> Data Type Conversion/1
  Compare To Zero/1 -> Logical Operator/1
  Relational Operator/1 -> Logical Operator/2
  Gain/1 -> Relational Operator/2
  hostVelocity/1 -> Gain/1
  message to speed limit conversion/1 -> Compare To Zero/1, Relational Operator/1
  MessageID/1 -> message to speed limit conversion/1
  Data Type Conversion/1 -> Warning/1

== system V2x_TC_CarBreakdownWarning_cs/Audi_A8_1/Traffic Controller/Traffic signs and  traffic lights controller/Enabled Subsystem/major object selection signs/If Action Subsystem/While Iterator Subsystem ==
  cond : Inport
  Compare To Zero : simulink/Logic and Bit Operations/Compare To Zero  SystemSampleTime=-1  relop===  LogicOutDataTypeMode=uint8  ZeroCross=off
  Selector : Selector  NumberOfDimensions=2  InputPortWidth=3  IndexOptions=Index vector (port),Index vector (dialog)  Indices=[1 3],1  OutputSizes=1,1
  While Iterator : WhileIterator  MaxIters=-1  WhileBlockType=do-while  ShowIterationPort=on  OutputDataType=double
  idx : Outport
  wires:
  Selector/1 -> Compare To Zero/1
  cond/1 -> Selector/1
  While Iterator/1 -> idx/1, Selector/2
  Compare To Zero/1 -> While Iterator/1

== system V2x_TC_CarBreakdownWarning_cs/Audi_A8_1/Traffic Controller/Intersection warning controller/Enabled Subsystem/Intersection/Intersection collision warning controller/For Each Subsystem/If Action Subsystem ==
  WM : Inport
  Rcross : Inport  Port=2
  target range : Inport  Port=3
  target angle : Inport  Port=4
  target intention : Inport  Port=5
  target heading : Inport  Port=6
  Action Port : ActionPort  ActionType=then
  Decision Algorithm : Stateflow chart  TreatAsAtomicUnit=on
  warning left lane : Outport  InitialOutput=false(1)
  warning straight lane : Outport  Port=2  InitialOutput=false(1)
  warning right lane : Outport  Port=3  InitialOutput=false(1)
  wires:
  Decision Algorithm/1(wLeft) -> warning left lane/1
  Rcross/1 -> Decision Algorithm/2(Rcross)
  target range/1 -> Decision Algorithm/3(range)
  Decision Algorithm/2(wStraight) -> warning straight lane/1
  target angle/1 -> Decision Algorithm/4(angle)
  target intention/1 -> Decision Algorithm/5(intention)
  Decision Algorithm/3(wRight) -> warning right lane/1
  target heading/1 -> Decision Algorithm/6(heading)
  WM/1 -> Decision Algorithm/1(WM)

== system V2x_TC_CarBreakdownWarning_cs/Audi_A8_1/Traffic Controller/Intersection warning controller/Enabled Subsystem/Intersection/Intersection collision warning controller/For Each Subsystem/If Action Subsystem1 ==
  Action Port : ActionPort  ActionType=else
  Constant : Constant  Value=false(1)
  Constant1 : Constant  Value=false(1)
  Constant2 : Constant  Value=false(1)
  warning left lane : Outport  InitialOutput=false(1)
  warning straight lane : Outport  Port=2  InitialOutput=false(1)
  warning right lane : Outport  Port=3  InitialOutput=false(1)
  wires:
  Constant/1 -> warning left lane/1
  Constant1/1 -> warning straight lane/1
  Constant2/1 -> warning right lane/1

== stateflow chart Audi_A8_1/Traffic Controller/Intersection warning controller/Enabled Subsystem/Intersection/Intersection collision warning controller/For Each Subsystem/If Action Subsystem/Decision Algorithm ==
  state controller
    state Lane3
      state Straight
        en: wRight=WM[8];
      state RightTurn
        en: wRight=WM[7];
      state LeftTurn
        en: wRight=WM[9];
      (junction 19) -> controller.Lane3.LeftTurn [order 2] : [intention<0]
      (junction 19) -> controller.Lane3.Straight [order 3] : [intention==0]
      (default) -> (junction 19) [order 1]
      (default) -> controller.Lane3.Straight [order 2]
      (junction 19) -> controller.Lane3.RightTurn [order 1] : [intention>0]
    state Lane2
      state RightTurn
        en: wStraight=WM[4];
      state LeftTurn
        en: wStraight=WM[6];
      state Straight
        en: wStraight=WM[5];
      (junction 18) -> controller.Lane2.Straight [order 2] : [intention==0]
      (default) -> controller.Lane2.Straight [order 2]
      (junction 18) -> controller.Lane2.RightTurn [order 3] : [intention>0]
      (junction 18) -> controller.Lane2.LeftTurn [order 1] : [intention<0]
      (default) -> (junction 18) [order 1]
    state Lane1
      state Straight
        en: wLeft=WM[2];
      state LeftTurn
        en: wLeft=WM[3];
      state RightTurn
        en: wLeft=WM[1];
      (junction 17) -> controller.Lane1.RightTurn [order 3] : [intention>0]
      (junction 17) -> controller.Lane1.LeftTurn [order 1] : [intention<0]
      (junction 17) -> controller.Lane1.Straight [order 2] : [intention==0]
      (default) -> controller.Lane1.Straight [order 2]
      (default) -> (junction 17) [order 1]
    state Enter
    controller.Lane1.LeftTurn -> Enter
    controller.Lane3.RightTurn -> Enter
    (default) -> Enter : {wLeft=0;
        | wStraight=0;
        | wRight=0;}
    controller.Lane3.Straight -> Enter
    controller.Lane3.LeftTurn -> Enter
    Enter -> Enter [order 4] : {wLeft=0;
        | wStraight=0;
        | wRight=0;}
    controller.Lane1.RightTurn -> Enter
    Enter -> Lane3 [order 2] : [angle>-90 && angle<-45 && range<Rcross...
        | && (heading>45 && heading<135)]
    controller.Lane1.Straight -> Enter
    controller.Lane2.RightTurn -> Enter
    controller.Lane2.LeftTurn -> Enter
    Enter -> Lane2 [order 1] : [angle>0 && angle<45 && range<Rcross...
        | && heading>135 && heading<225]
    Enter -> Lane1 [order 3] : [angle>90 && angle<135 && range<Rcross...
        | && heading>225 && heading<315]
    controller.Lane2.Straight -> Enter
  data: WM input double size=9; Rcross input double; range input double; angle input double; intention input double; heading input double; wLeft output boolean size=1 =false(1); wStraight output boolean size=1 =false(1); wRight output boolean size=1 =false(1)

== matlab function Audi_A8_1/Traffic Controller/Intersection warning controller/Enabled Subsystem/sort using ID/Embedded MATLAB Function ==
  data: y output double; ids input double
function y = fcn(ids)
% Sorts ID vector

[~,y] = sort(ids,'descend');

end

== matlab function Audi_A8_1/Rx_Noise/Embedded MATLAB Function ==
  data: CAM_warning input double; CAM output double; CAM_messageID input double; CAM_vehicleID input double; CAM_vehicleType input double; CAM_publicVehicleType input double; CAM_lightBarInUse input double; CAM_sireneInUse input double; CAM_velocity input double; CAM_acceleration input double; CAM_yawRate input double; CAM_turnAdvice input double; CAM_trafficLightPriority input double; CAM_GPSlat input double; CAM_GPSlong input double; CAM_GPSalt input double; CAM_rotZ input double
function CAM = fcn(CAM_warning, CAM_messageID, CAM_vehicleID, CAM_vehicleType, CAM_publicVehicleType, CAM_lightBarInUse, CAM_sireneInUse, CAM_velocity, CAM_acceleration, CAM_yawRate, CAM_turnAdvice, CAM_trafficLightPriority, CAM_GPSlat, CAM_GPSlong, CAM_GPSalt, CAM_rotZ)
%#eml

CAM = [CAM_warning, CAM_messageID, CAM_vehicleID, CAM_vehicleType, CAM_publicVehicleType, CAM_lightBarInUse, CAM_sireneInUse, CAM_velocity, CAM_acceleration, CAM_yawRate, CAM_turnAdvice, CAM_trafficLightPriority, CAM_GPSlat, CAM_GPSlong, CAM_GPSalt, CAM_rotZ];

== matlab function Audi_A8_1/Rx_Noise/Embedded MATLAB Function1 ==
  data: CAM_warning output double; CAM input double; CAM_messageID output double; CAM_vehicleID output double; CAM_vehicleType output double; CAM_publicVehicleType output double; CAM_lightBarInUse output double; CAM_sireneInUse output double; CAM_velocity output double; CAM_acceleration output double; CAM_yawRate output double; CAM_turnAdvice output double; CAM_trafficLightPriority output double; CAM_GPSlat output double; CAM_GPSlong output double; CAM_GPSalt output double; CAM_rotZ output double
function [CAM_warning, CAM_messageID, CAM_vehicleID, CAM_vehicleType, CAM_publicVehicleType, CAM_lightBarInUse, CAM_sireneInUse, CAM_velocity, CAM_acceleration, CAM_yawRate, CAM_turnAdvice, CAM_trafficLightPriority, CAM_GPSlat, CAM_GPSlong, CAM_GPSalt, CAM_rotZ] = fcn(CAM)
%#eml

CAM_warning = CAM(:, 1);
CAM_messageID = CAM(:, 2); 
CAM_vehicleID = CAM(:, 3);
CAM_vehicleType = CAM(:, 4);
CAM_publicVehicleType = CAM(:, 5);
CAM_lightBarInUse = CAM(:, 6);
CAM_sireneInUse = CAM(:, 7);
CAM_velocity = CAM(:, 8);
CAM_acceleration = CAM(:, 9);
CAM_yawRate = CAM(:, 10);
CAM_turnAdvice = CAM(:, 11);
CAM_trafficLightPriority = CAM(:, 12);
CAM_GPSlat = CAM(:, 13);
CAM_GPSlong = CAM(:, 14);
CAM_GPSalt = CAM(:, 15);
CAM_rotZ = CAM(:, 16);
